simulink model "Offline_LQG"  (R2022b)
settings: Solver=ode45  StartTime=0.0  StopTime=30  RelTol=1e-3
undefined symbols (not defined in the file): A, B, C, D, delta_x0_hat, K_lqeta, K_lqx, L_kf, voltage_max
settings Model: Creator=fabio  LastModifiedBy=utente
settings SolverCC: AlgebraicLoopSolver=TrustRegion
settings OptimizationCC: BlockReduction=off  DefaultParameterBehavior=Inlined  BufferReuse=off
settings DebuggingCC: UnconnectedInputMsg=warning  UnconnectedOutputMsg=warning  SFMachineParentedDataDiag=warning
settings ModelReferenceCC: EnableRefExpFcnMdlSchedulingChecks=on
settings RTWCC: DLArmComputeVersion=19.05

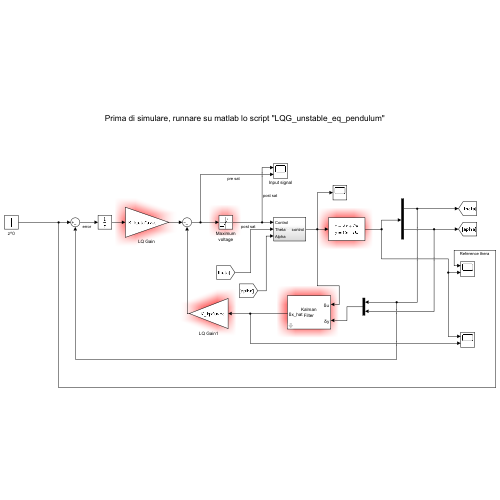
[thumbnail: Simulink's stored preview of the top-level diagram]
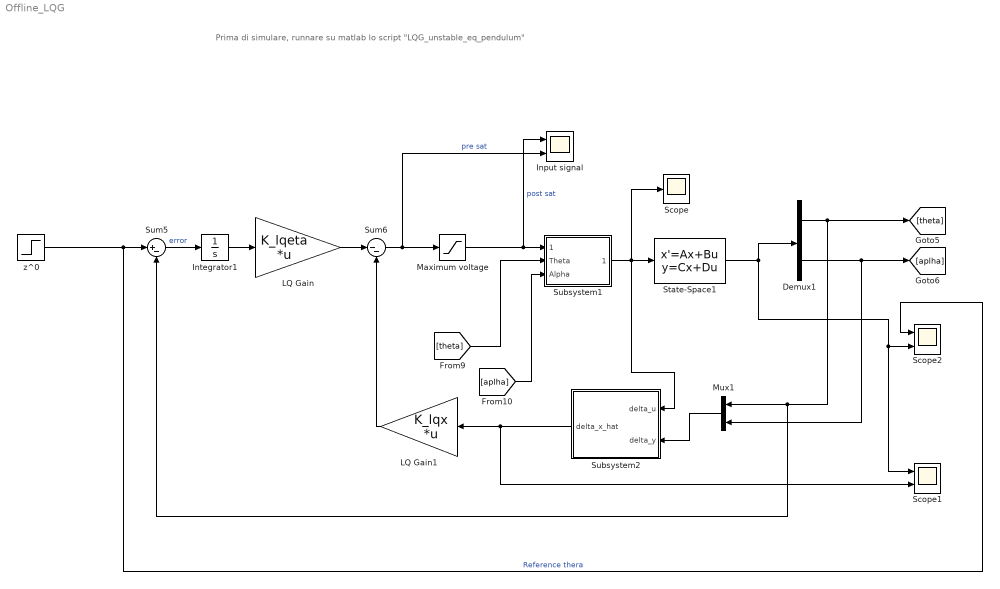
== system Offline_LQG ==
  note: Prima di simulare, runnare su matlab lo script "LQG_unstable_eq_pendulum"
  Demux1 : Demux  Outputs=2
  Input signal : Scope  NumInputPorts=2
  Integrator1 : Integrator
  "LQ Gain " : Gain  Gain=K_lqeta  Multiplication=Matrix(K*u) (u vector)
  LQ Gain1 : Gain  Gain=K_lqx  Multiplication=Matrix(K*u) (u vector)
  Maximum voltage : Saturate  UpperLimit=voltage_max  LowerLimit=-voltage_max
  Mux1 : Mux  Inputs=2
  Scope : Scope
  Scope1 : Scope  NumInputPorts=2
  Scope2 : Scope  NumInputPorts=2
  State-Space1 : StateSpace  A=A  B=B  C=C  D=D  InitialCondition=[0 0 0 0]
  Subsystem1 : Subsystem
  Subsystem2 : Subsystem  mask(Continuous time Kalman Filter){A_sys=A, B_sys=B, C_sys=C, D_sys=D, L=L_kf, x0_hat=delta_x0_hat}
      mask prompts: A_sys "A:"; B_sys "B:"; C_sys "C:"; D_sys "D:"; L "Gain"; x0_hat "Initial guess"
      mask DialogControl ParameterGroupVar Prompt: System parameters
      mask Display:
      | disp('Kalman\nFilter');
      | port_label('input', 1, '{\delta}u', 'interpreter', 'tex');
      | port_label('input', 2, '{\delta}y', 'interpreter', 'tex');
      | port_label('output', 1, '{\delta}x\_hat', 'interpreter', 'tex');
  Sum5 : Sum  Inputs=|+-
  Sum6 : Sum  Inputs=|--
  z^0 : Step  Time=5  After=0.3  SampleTime=0
  wires:
  z^0/1 -> Scope2/1, Sum5/1  "Reference thera"
  "LQ Gain "/1 -> Sum6/1
  LQ Gain1/1 -> Sum6/2
  Demux1/2 -> Mux1/2, [aplha]
  Integrator1/1 -> "LQ Gain "/1
  Demux1/1 -> Mux1/1, Sum5/2, [theta]
  Maximum voltage/1 -> Input signal/1, Subsystem1/1(Control)  "post sat"
  Subsystem1/1(control) -> State-Space1/1, Subsystem2/1(delta_u), Scope/1
  State-Space1/1 -> Scope1/1, Scope2/2, Demux1/1
  [aplha] -> Subsystem1/3(Alpha)
  Sum5/1 -> Integrator1/1  "error"
  [theta] -> Subsystem1/2(Theta)
  Sum6/1 -> Input signal/2, Maximum voltage/1  "pre sat"
  Mux1/1 -> Subsystem2/2(delta_y)
  Subsystem2/1(delta_x_hat) -> Scope1/2, LQ Gain1/1

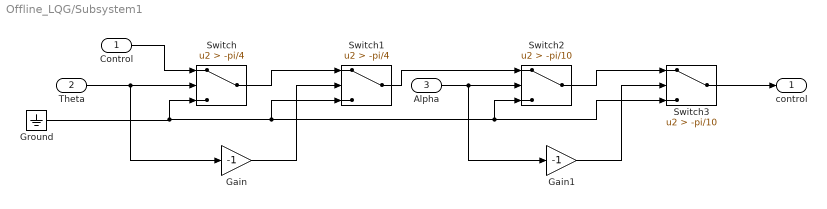
== system Offline_LQG/Subsystem1 ==
  Control : Inport
  Theta : Inport  Port=2
  Alpha : Inport  Port=3
  Gain : Gain  Gain=-1
  Gain1 : Gain  Gain=-1
  Ground : Ground
  Switch : Switch  Criteria=u2 > Threshold  Threshold=-pi/4  SaturateOnIntegerOverflow=off  InputSameDT=off
  Switch1 : Switch  Criteria=u2 > Threshold  Threshold=-pi/4  SaturateOnIntegerOverflow=off  InputSameDT=off
  Switch2 : Switch  Criteria=u2 > Threshold  Threshold=-pi/10  SaturateOnIntegerOverflow=off  InputSameDT=off
  Switch3 : Switch  Criteria=u2 > Threshold  Threshold=-pi/10  SaturateOnIntegerOverflow=off  InputSameDT=off
  control : Outport
  wires:
  Gain/1 -> Switch1/2
  Theta/1 -> Gain/1, Switch/2
  Control/1 -> Switch/1
  Switch/1 -> Switch1/1
  Gain1/1 -> Switch3/2
  Switch1/1 -> Switch2/1
  Ground/1 -> Switch3/3, Switch2/3, Switch1/3, Switch/3
  Switch2/1 -> Switch3/1
  Alpha/1 -> Switch2/2, Gain1/1
  Switch3/1 -> control/1

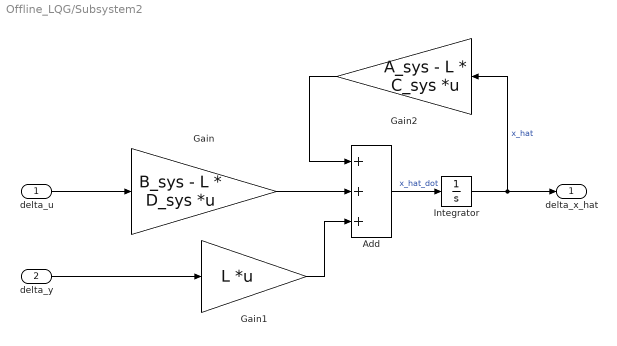
== system Offline_LQG/Subsystem2 ==
  delta_u : Inport  PortDimensions=1
  delta_y : Inport  Port=2  PortDimensions=2
  Add : Sum  Inputs=+++
  Gain : Gain  Gain=B_sys - L * D_sys  Multiplication=Matrix(K*u) (u vector)
  Gain1 : Gain  Gain=L  Multiplication=Matrix(K*u) (u vector)
  Gain2 : Gain  Gain=A_sys - L * C_sys  Multiplication=Matrix(K*u) (u vector)
  Integrator : Integrator
  delta_x_hat : Outport  PortDimensions=4
  wires:
  delta_u/1 -> Gain/1
  Gain/1 -> Add/2
  delta_y/1 -> Gain1/1
  Add/1 -> Integrator/1  "x_hat_dot"
  Integrator/1 -> Gain2/1, delta_x_hat/1  "x_hat"
  Gain2/1 -> Add/1
  Gain1/1 -> Add/3
